simulink subsystem "AdaptadorSonarLeds"  (R2021b)
settings: Solver=VariableStepAuto  StartTime=0.0  StopTime=10.0  RelTol=1e-3
libraries: simulink x2
settings Model: Creator=Mauri  LastModifiedBy=yo

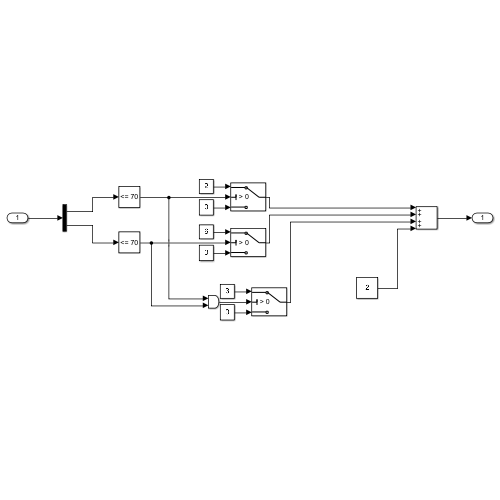
[thumbnail: Simulink's stored preview of the top-level diagram]
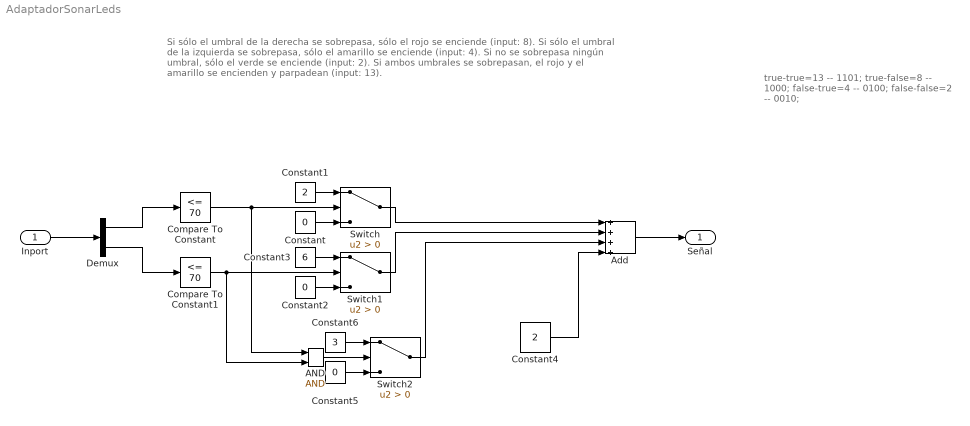
== system AdaptadorSonarLeds ==
  note: Si sólo el umbral de la derecha se sobrepasa, sólo el rojo se enciende (input: 8). Si sólo el umbral de la izquierda se sobrepasa, sólo el amarillo se enciende (input: 4). Si no se sobrepasa ningún umbral, sólo el verde se enciende (input: 2). Si ambos umbrales se sobrepasan, el rojo y el amarillo se encienden y parpadean (input: 13).
  note: true-true=13 -- 1101;
      | true-false=8 -- 1000;
      | false-true=4 -- 0100;
      | false-false=2 -- 0010;
  Inport : Inport
  AND : Logic  IconShape=distinctive  AllPortsSameDT=off  OutDataTypeStr=boolean
  Add : Sum  Inputs=++++  AccumDataTypeStr=uint8  OutDataTypeStr=uint8
  Compare To Constant : simulink/Logic and Bit Operations/Compare To Constant  relop=<=  const=70  OutDataTypeStr=boolean
  Compare To Constant1 : simulink/Logic and Bit Operations/Compare To Constant  relop=<=  const=70  OutDataTypeStr=boolean
  Constant : Constant  Value=0
  Constant1 : Constant  Value=2  OutDataTypeStr=uint8
  Constant2 : Constant  Value=0
  Constant3 : Constant  Value=6  OutDataTypeStr=uint8
  Constant4 : Constant  Value=2  OutDataTypeStr=uint8
  Constant5 : Constant  Value=0
  Constant6 : Constant  Value=3  OutDataTypeStr=uint8
  Demux : Demux  Outputs=2
  Switch : Switch  Criteria=u2 > Threshold
  Switch1 : Switch  Criteria=u2 > Threshold
  Switch2 : Switch  Criteria=u2 > Threshold
  Señal : Outport
  wires:
  Inport/1 -> Demux/1
  Constant1/1 -> Switch/1
  Constant/1 -> Switch/3
  Demux/1 -> Compare To Constant/1
  Compare To Constant/1 -> Switch/2, AND/1
  Constant2/1 -> Switch1/3
  Constant3/1 -> Switch1/1
  Compare To Constant1/1 -> Switch1/2, AND/2
  Demux/2 -> Compare To Constant1/1
  Add/1 -> Señal/1
  Constant4/1 -> Add/4
  Switch/1 -> Add/1
  Switch1/1 -> Add/2
  Constant5/1 -> Switch2/3
  AND/1 -> Switch2/2
  Constant6/1 -> Switch2/1
  Switch2/1 -> Add/3
